simulink subsystem "ControladorBorroso_parte1"  (R2019b)
settings: Solver=VariableStepAuto  StartTime=0.0  StopTime=10.0  RelTol=1e-3
libraries: fuzblock x1, simulink x1
settings Model: Creator=laura  LastModifiedBy=laura

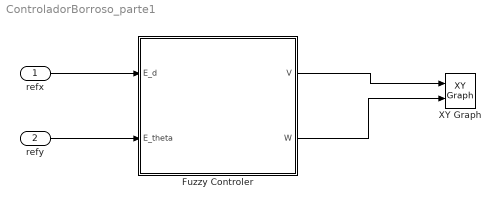
== system ControladorBorroso_parte1 ==
  "refx " : Inport
  refy : Inport  Port=2
  Fuzzy Controler : Subsystem
  XY Graph : simulink/Sinks/XY Graph  xmin=-5  xmax=5  ymin=-5  ymax=5  st=-1
  wires:
  "refx "/1 -> Fuzzy Controler/1("E_d ")
  refy/1 -> Fuzzy Controler/2("E_theta ")
  Fuzzy Controler/1(V) -> XY Graph/1
  Fuzzy Controler/2(W) -> XY Graph/2

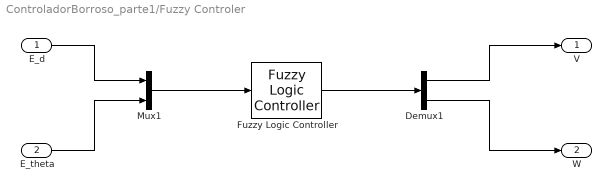
== system ControladorBorroso_parte1/Fuzzy Controler ==
  "E_d " : Inport
  "E_theta " : Inport  Port=2
  Demux1 : Demux  Outputs=2
  Fuzzy Logic Controller : fuzblock/Fuzzy Logic  Controller  FIS='ControlBorroso1.fis'  OutputSampleNumber=101  DataType=double  FuzzifiedInputs=off  RuleFiringStrengths=off  RuleOutputs=off  AggregatedOutputs=off  SimulateUsing=Interpreted execution  OutOfRangeInputValueMessage=warning  NoRuleFiredMessage=warning  EmptyOutputFuzzySetMessage=warning
  Mux1 : Mux  Inputs=2
  V : Outport
  W : Outport  Port=2
  wires:
  Fuzzy Logic Controller/1 -> Demux1/1
  "E_theta "/1 -> Mux1/2
  Demux1/2 -> W/1
  Demux1/1 -> V/1
  "E_d "/1 -> Mux1/1
  Mux1/1 -> Fuzzy Logic Controller/1
